simulink model "TidalTurbine"  (R2025b)
settings: Solver=VariableStepAuto  StartTime=0.0  StopTime=10.0  RelTol=1e-3
values from neighbouring files (symbols this model uses):
  A = pi * 10^2    (= 314.159265359)    [TidalTurbinePower.m]
  Cp = 0.35    [TidalTurbinePower.m]
  g = 9.81    [TidalTurbinePower.m]
  rho = 1000    [TidalTurbinePower.m]
settings Model: Creator=rvdjo  LastModifiedBy=rvdjo

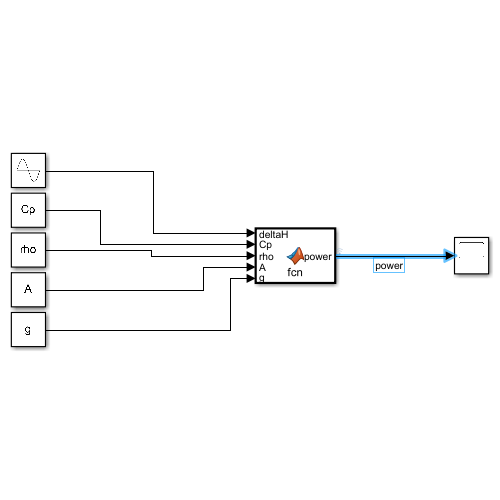
[thumbnail: Simulink's stored preview of the top-level diagram]
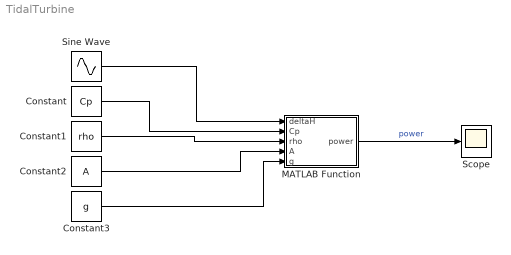
== system TidalTurbine ==
  Constant : Constant  Value=Cp
  Constant1 : Constant  Value=rho
  Constant2 : Constant  Value=A
  Constant3 : Constant  Value=g
  MATLAB Function : MATLAB Function  TreatAsAtomicUnit=on
  Scope : Scope
      settings: ActiveDisplayYMinimum=-387668.48945610283  ActiveDisplayYMaximum=3.4890164051049259E+6
  Sine Wave : Sin  Amplitude=0.75  SampleTime=0
  wires:
  Sine Wave/1 -> MATLAB Function/1(deltaH)
  MATLAB Function/1(power) -> Scope/1  "power"
  Constant/1 -> MATLAB Function/2(Cp)
  Constant1/1 -> MATLAB Function/3(rho)
  Constant2/1 -> MATLAB Function/4(A)
  Constant3/1 -> MATLAB Function/5(g)

== matlab function TidalTurbine/MATLAB Function ==
  data: power output; deltaH input; Cp input; rho input; A input; g input
%% Power Output from a Tidal Turbine

% The Sine Wave block in the model represents the height differential, ΔH, 
% of the water on different sides of the turbine.

function power = fcn(deltaH,Cp,rho,A,g) % deltaH = ΔH

% Equation for power
power = 0.5 * Cp * rho * A * (2 * g * abs(deltaH)) ^ (1.5);
